simulink model "ideal_buck_boost"  (R2018a)
settings: Solver=VariableStepAuto  StartTime=0.0  StopTime=0.2  RelTol=1e-3
undefined symbols (not defined in the file): A, B, Co, current_correction_start, disturbance_Ro_enable, disturbance_Ro_time, disturbance_Vin_enable, disturbance_Vin_time, Fsw, L, opt_constant_reference, opt_equilibrium_controller, opt_pwm, opt_pwm_current_controller, opt_theorem, opt_update_equilibrium, P, pwm_limit_lower, pwm_limit_upper, pwm_period, pwm_pid_kd, pwm_pid_ki, pwm_pid_kp, pwm_pid_vc_ci, pwm_pid_vc_cp, pwm_pid_vc_vi, pwm_pid_vc_vp, pwm_sample_time, Q, R, reference_controller_initial, reference_pid_ki, reference_pid_kp, Ro, Ro_p, sys, tau, Ti, ts, Vo, Vs, Vs_p, xe
libraries: powerlib x17, simulink x12, pePwmGenerator x2
settings Model: Creator=TARCIO-FEM  LastModifiedBy=Julio-LEPO
settings OptimizationCC: EfficientMapNaN2IntZero=off
settings HardwareCC: TargetBitPerPointer=64  TargetBitPerSizeT=64  TargetBitPerPtrDiffT=64  TargetLongLongMode=on  TargetIntDivRoundTo=Zero  TargetEndianess=LittleEndian  TargetWordSize=64  TargetHWDeviceType=MATLAB Host  ProdEqTarget=off
settings CodeAppCC: MaxIdLength=128
settings GRTTargetCC: TargetLangStandard=C89/C90 (ANSI)  CombineOutputUpdateFcns=off  GRTInterface=on

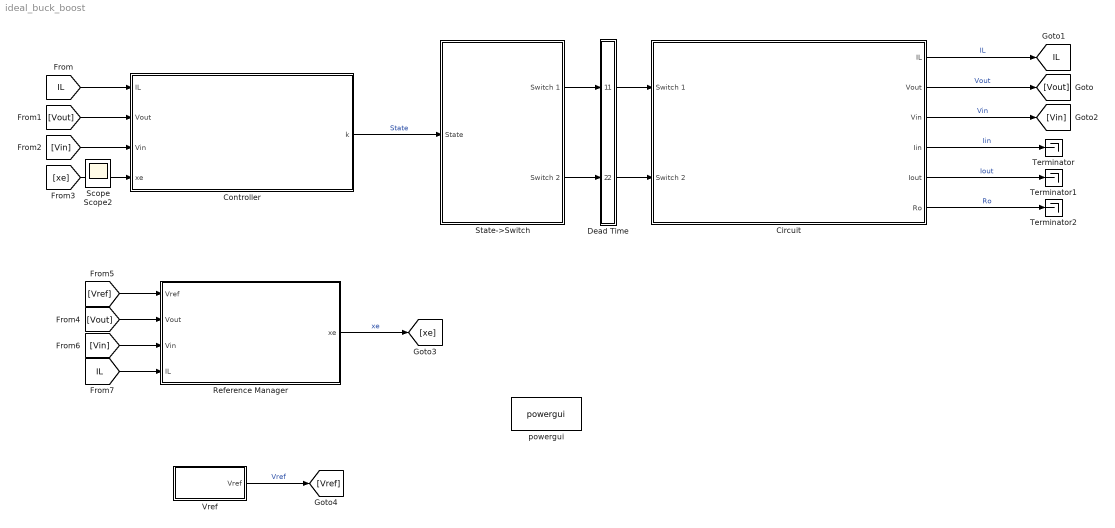
== system ideal_buck_boost ==
  Circuit : Subsystem
  Controller : Subsystem
  Dead Time : Subsystem
  Reference Manager : Subsystem
  State->Switch : Subsystem
  Terminator : Terminator
  Terminator1 : Terminator
  Terminator2 : Terminator
  Vref : Subsystem
  powergui : powerlib/powergui  Priority=1  SimulationMode=Discrete  SampleTime=Ti  frequency=60  Iterations=50  frequencyindice=0  Pbase=100e6  ErrMax=1e-4  UnitsV=kV  UnitsW=MW  buscounter=0  FunctionMessages=off  echomessages=off  EnableUseOfTLC=off  CurrentSourceSwitches=off  DisableSnubberDevices=off  DisableRonSwitches=off  DisableVfSwitches=off  DisplayEquations=off  SolverType=Tustin/Backward Euler (TBE)  Interpol=off  ExternalGateDelay=off  methode=off  Ts=100  x0status=blocks  SPID=on  SwTol=0  HookPort=off  RestoreLinks=warning  ResistiveCurrentMeasurement=off  Frange=[0:2:500]  Ylog=off  Xlog=on  ShowGrid=off  save=off  variable=ZData  structure=0  ZoomFFT=off  StartTime=0.0  cycles=1  DisplayStyle=1  fundamental=60  FreqAxis=off  MaxFrequency=1000  frequencyindicesteady=1  RmsSteady=1  display=off
  Scope : Scope
  Scope2 : Scope
  tag scope: IL=global
  wires:
  Controller/1(k) -> State->Switch/1(State)  "State"
  Circuit/3(Vin) -> [Vin]  "Vin"
  Circuit/5(Iout) -> Terminator1/1  "Iout"
  Circuit/4(Iin) -> Terminator/1  "Iin"
  Circuit/2(Vout) -> [Vout]  "Vout"
  Circuit/1(IL) -> [IL]  "IL"
  [Vout] -> Reference Manager/2(Vout)
  [Vref] -> Reference Manager/1(Vref)
  [Vin] -> Reference Manager/3(Vin)
  [IL] -> Reference Manager/4(IL)
  Reference Manager/1(xe) -> [xe]  "xe"
  Vref/1(Vref) -> [Vref]  "Vref"
  Circuit/6(Ro) -> Terminator2/1  "Ro"
  [Vout] -> Controller/2(Vout)
  [xe] -> Controller/4(xe)
  [Vin] -> Controller/3(Vin)
  [IL] -> Controller/1(IL)
  State->Switch/2(Switch 2) -> Dead Time/2(In2)
  State->Switch/1(Switch 1) -> Dead Time/1(In1)
  Dead Time/1(Out1) -> Circuit/1(Switch 1)
  Dead Time/2(Out2) -> Circuit/2(Switch 2)

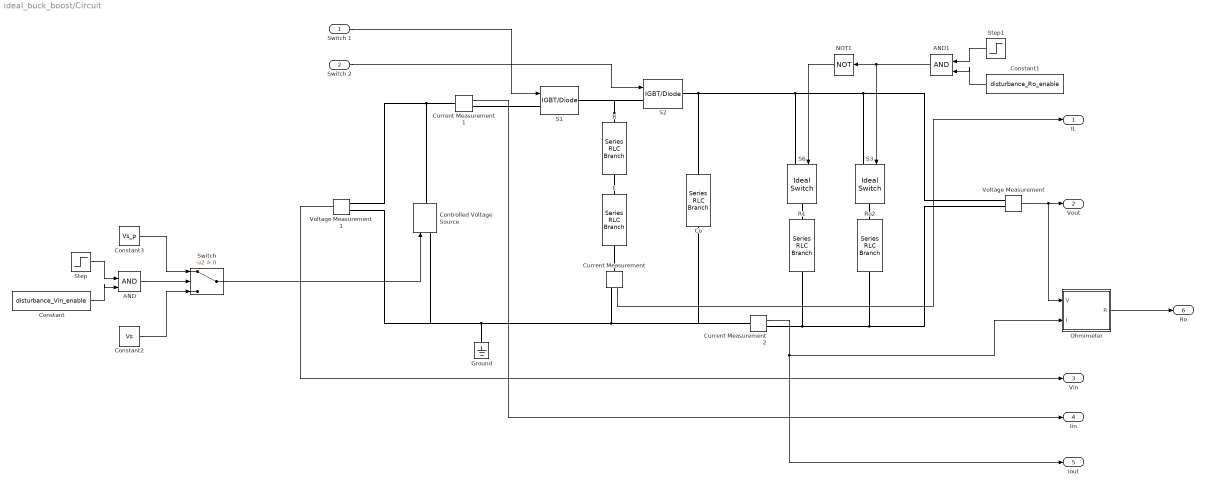
== system ideal_buck_boost/Circuit ==
  Switch 1 : Inport
  Switch 2 : Inport  Port=2
  AND : Logic  IconShape=distinctive  AllPortsSameDT=off  OutDataTypeStr=boolean
  AND1 : Logic  IconShape=distinctive  AllPortsSameDT=off  OutDataTypeStr=boolean
  Co : powerlib/Elements/Series RLC Branch  LConnTagsString=__new0  RConnTagsString=__new0  BranchType=C  Resistance=1  Inductance=L  SetiL0=off  InitialCurrent=0  Capacitance=Co  Setx0=off  InitialVoltage=0  Measurements=None
  Constant : Constant  Value=disturbance_Vin_enable
  Constant1 : Constant  Value=disturbance_Ro_enable
  Constant2 : Constant  Value=Vs
  Constant3 : Constant  Value=Vs_p
  Controlled Voltage Source : powerlib/Electrical Sources/Controlled Voltage Source  Initialize=on  Source_Type=DC  Amplitude=0  Phase=0  Frequency=0  Measurements=None
  Current Measurement : powerlib/Measurements/Current Measurement  PhasorSimulation=off  OutputType=Complex  PSBequivalent=0
  Current Measurement1 : powerlib/Measurements/Current Measurement  PhasorSimulation=off  OutputType=Complex  PSBequivalent=0
  Current Measurement2 : powerlib/Measurements/Current Measurement  PhasorSimulation=off  OutputType=Complex  PSBequivalent=0
  Ground : powerlib/Elements/Ground  LConnTagsString=a
  L : powerlib/Elements/Series RLC Branch  LConnTagsString=__new0  RConnTagsString=__new0  BranchType=L  Resistance=1  Inductance=L  SetiL0=off  InitialCurrent=0  Capacitance=1e-6  Setx0=off  InitialVoltage=0  Measurements=None
  NOT1 : Logic  Operator=NOT  IconShape=distinctive  AllPortsSameDT=off  OutDataTypeStr=boolean
  Ohmimeter : Subsystem
  R : powerlib/Elements/Series RLC Branch  LConnTagsString=__new0  RConnTagsString=__new0  BranchType=R  Resistance=R  Inductance=1e-3  SetiL0=off  InitialCurrent=0  Capacitance=1e-6  Setx0=off  InitialVoltage=0  Measurements=None
  R1 : powerlib/Elements/Series RLC Branch  LConnTagsString=__new0  RConnTagsString=__new0  BranchType=R  Resistance=Ro  Inductance=1e-3  SetiL0=off  InitialCurrent=0  Capacitance=1e-6  Setx0=off  InitialVoltage=0  Measurements=None
  Ro2 : powerlib/Elements/Series RLC Branch  LConnTagsString=__new0  RConnTagsString=__new0  BranchType=R  Resistance=Ro_p  Inductance=1e-3  SetiL0=off  InitialCurrent=0  Capacitance=1e-6  Setx0=off  InitialVoltage=0  Measurements=None
  S1 : powerlib/Power Electronics/IGBT//Diode  Ron=1e-3  Rs=1e5  Cs=inf  Measurements=off
  S2 : powerlib/Power Electronics/IGBT//Diode  Ron=1e-3  Rs=1e5  Cs=inf  Measurements=off
  S3 : powerlib/Power Electronics/Ideal Switch  Ron=0.001  Lon=0  IC=0  Rs=1e5  Cs=inf  Measurements=off
  S6 : powerlib/Power Electronics/Ideal Switch  Ron=0.001  Lon=0  IC=0  Rs=1e5  Cs=inf  Measurements=off
  Step : Step  Time=disturbance_Vin_time  SampleTime=0
  Step1 : Step  Time=disturbance_Ro_time  SampleTime=0
  Switch : Switch  Criteria=u2 > Threshold
  Voltage Measurement : powerlib/Measurements/Voltage Measurement  PhasorSimulation=off  OutputType=Complex  PSBequivalent=0
  Voltage Measurement1 : powerlib/Measurements/Voltage Measurement  PhasorSimulation=off  OutputType=Complex  PSBequivalent=0
  IL : Outport
  Vout : Outport  Port=2
  Vin : Outport  Port=3
  Iin : Outport  Port=4
  Iout : Outport  Port=5
  Ro : Outport  Port=6
  wires:
  Switch 1/1 -> S1/1
  Voltage Measurement1/1 -> Vin/1
  Current Measurement/1 -> IL/1
  Voltage Measurement/1 -> Ohmimeter/1(V), Vout/1
  Switch 2/1 -> S2/1
  AND/1 -> Switch/2
  Constant/1 -> AND/2
  Switch/1 -> Controlled Voltage Source/1
  Step/1 -> AND/1
  Constant2/1 -> Switch/3
  Constant3/1 -> Switch/1
  NOT1/1 -> S6/1
  Constant1/1 -> AND1/2
  AND1/1 -> S3/1, NOT1/1
  Step1/1 -> AND1/1
  Current Measurement1/1 -> Iin/1
  Current Measurement2/1 -> Ohmimeter/2(I), Iout/1
  Ohmimeter/1(R) -> Ro/1
  connections:
  L/LConn1 -- R/RConn1
  R/LConn1 -- S2/LConn1 -- S1/RConn1
  Current Measurement/LConn1 -- L/RConn1
  Controlled Voltage Source/RConn1 -- Current Measurement1/LConn1 -- Voltage Measurement1/LConn1
  S6/LConn1 -- S2/RConn1 -- Co/RConn1 -- S3/LConn1 -- Voltage Measurement/LConn2
  Ground/LConn1 -- Current Measurement/RConn1 -- Co/LConn1 -- Current Measurement2/LConn1 -- Voltage Measurement1/LConn2 -- Controlled Voltage Source/LConn1
  S3/RConn1 -- Ro2/LConn1
  S6/RConn1 -- R1/LConn1
  S1/LConn1 -- Current Measurement1/RConn1
  R1/RConn1 -- Current Measurement2/RConn1 -- Voltage Measurement/LConn1 -- Ro2/RConn1

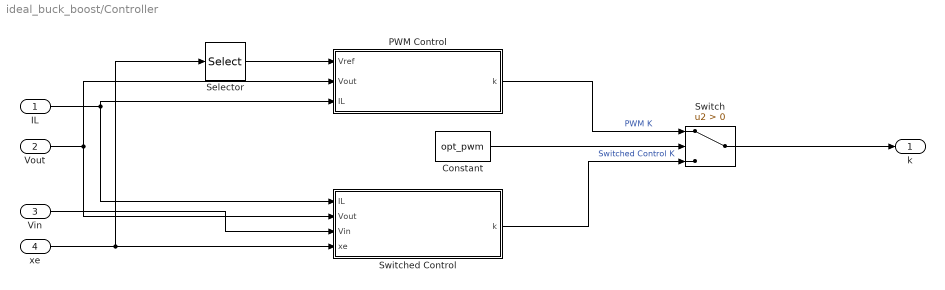
== system ideal_buck_boost/Controller ==
  IL : Inport
  Vout : Inport  Port=2
  Vin : Inport  Port=3
  xe : Inport  Port=4
  Constant : Constant  Value=opt_pwm
  PWM Control : Subsystem
  Selector : Selector  InputPortWidth=2  IndexOptions=Index vector (dialog)  Indices=[2]  OutputSizes=1
  Switch : Switch  Criteria=u2 > Threshold
  Switched Control : Subsystem
  k : Outport
  wires:
  IL/1 -> PWM Control/3(IL), Switched Control/1(IL)
  Vout/1 -> PWM Control/2(Vout), Switched Control/2(Vout)
  Vin/1 -> Switched Control/3(Vin)
  PWM Control/1(k) -> Switch/1  "PWM K"
  Switched Control/1(k) -> Switch/3  "Switched Control K"
  Constant/1 -> Switch/2
  xe/1 -> Selector/1, Switched Control/4(xe)
  Selector/1 -> PWM Control/1(Vref)
  Switch/1 -> k/1

== system ideal_buck_boost/Dead Time ==
  In1 : Inport
  In2 : Inport  Port=2
  Dead Time : Subsystem
  Dead Time1 : Subsystem
  Out1 : Outport
  Out2 : Outport  Port=2
  wires:
  Dead Time1/1(Signal Delayed) -> Out2/1
  In1/1 -> Dead Time/1(Signal)
  Dead Time/1(Signal Delayed) -> Out1/1
  In2/1 -> Dead Time1/1(Signal)

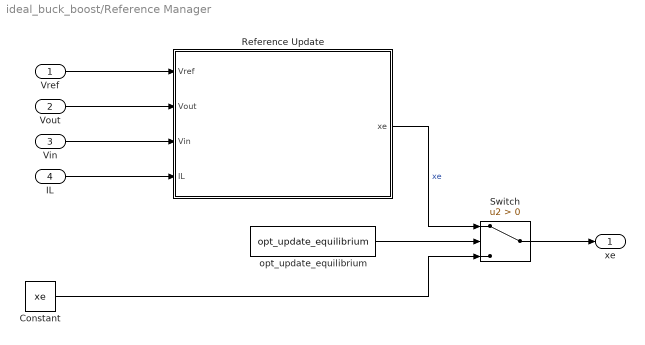
== system ideal_buck_boost/Reference Manager ==
  Vref : Inport
  Vout : Inport  Port=2
  Vin : Inport  Port=3
  IL : Inport  Port=4
  Constant : Constant  Value=xe
  Reference Update : Subsystem
  Switch : Switch  Criteria=u2 > Threshold
  opt_update_equilibrium : Constant  Value=opt_update_equilibrium
  xe : Outport
  wires:
  Vout/1 -> Reference Update/2(Vout)
  Vin/1 -> Reference Update/3(Vin)
  Vref/1 -> Reference Update/1(Vref)
  opt_update_equilibrium/1 -> Switch/2
  Switch/1 -> xe/1
  Reference Update/1(xe) -> Switch/1  "xe"
  Constant/1 -> Switch/3
  IL/1 -> Reference Update/4(IL)

== system ideal_buck_boost/State->Switch ==
  State : Inport
  Compare To Constant : simulink/Logic and Bit Operations/Compare To Constant  relop=<=  const=1.5  OutDataTypeStr=boolean
  NOT : Logic  Operator=NOT  IconShape=distinctive  AllPortsSameDT=off  OutDataTypeStr=boolean
  Switch 1 : Outport
  Switch 2 : Outport  Port=2
  wires:
  Compare To Constant/1 -> Switch 1/1, NOT/1  "Switch Signal"
  State/1 -> Compare To Constant/1
  NOT/1 -> Switch 2/1

== system ideal_buck_boost/Vref ==
  Constant Reference : Subsystem
  Switch1 : Switch  Criteria=u2 > Threshold
  Variable Reference : Subsystem
  opt_constant_reference : Constant  Value=opt_constant_reference
  Vref : Outport
  wires:
  opt_constant_reference/1 -> Switch1/2
  Switch1/1 -> Vref/1
  Variable Reference/1(Vref) -> Switch1/3
  Constant Reference/1(Vref) -> Switch1/1

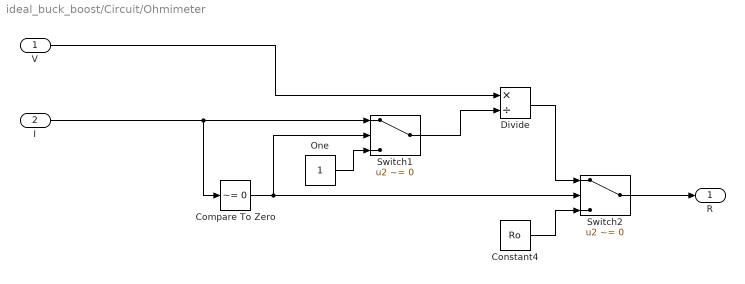
== system ideal_buck_boost/Circuit/Ohmimeter ==
  V : Inport
  I : Inport  Port=2
  Compare To Zero : simulink/Logic and Bit Operations/Compare To Zero  relop=~=  OutDataTypeStr=boolean
  Constant4 : Constant  Value=Ro
  Divide : Product  Inputs=*/
  One : Constant
  Switch1 : Switch  Criteria=u2 ~= 0
  Switch2 : Switch  Criteria=u2 ~= 0
  R : Outport
  wires:
  Compare To Zero/1 -> Switch1/2, Switch2/2
  I/1 -> Switch1/1, Compare To Zero/1
  Divide/1 -> Switch2/1
  Constant4/1 -> Switch2/3
  Switch1/1 -> Divide/2
  One/1 -> Switch1/3
  V/1 -> Divide/1
  Switch2/1 -> R/1

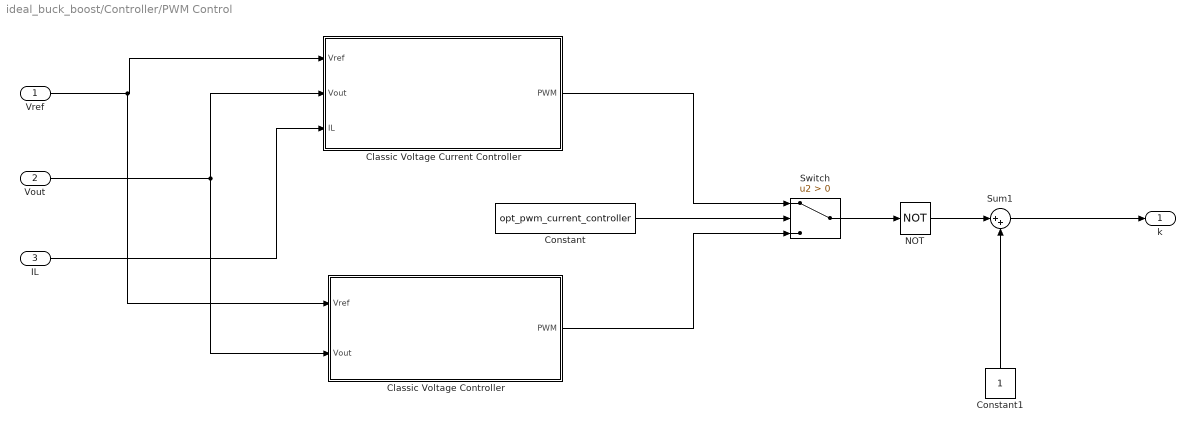
== system ideal_buck_boost/Controller/PWM Control ==
  Vref : Inport
  Vout : Inport  Port=2
  IL : Inport  Port=3
  Classic Voltage Controller : Subsystem
  Classic Voltage Current Controller : Subsystem
  Constant : Constant  Value=opt_pwm_current_controller
  Constant1 : Constant
  NOT : Logic  Operator=NOT  IconShape=distinctive  AllPortsSameDT=off  OutDataTypeStr=boolean
  Sum1 : Sum  Inputs=|++
  Switch : Switch  Criteria=u2 > Threshold
  k : Outport
  wires:
  Sum1/1 -> k/1
  NOT/1 -> Sum1/1
  Constant1/1 -> Sum1/2
  Vref/1 -> Classic Voltage Controller/1(Vref), Classic Voltage Current Controller/1(Vref)
  Vout/1 -> Classic Voltage Controller/2(Vout), Classic Voltage Current Controller/2(Vout)
  IL/1 -> Classic Voltage Current Controller/3(IL)
  Constant/1 -> Switch/2
  Switch/1 -> NOT/1
  Classic Voltage Controller/1(PWM) -> Switch/3
  Classic Voltage Current Controller/1(PWM) -> Switch/1

== system ideal_buck_boost/Controller/Switched Control ==
  IL : Inport
  Vout : Inport  Port=2
  Vin : Inport  Port=3
  xe : Inport  Port=4
  Mux : Mux  Inputs=2
  Switching Strategy : MATLAB Function  TreatAsAtomicUnit=on
  System Properties : Subsystem
  Zero-Order Hold : ZeroOrderHold  SampleTime=1/Fsw
  k : Outport
  wires:
  Vin/1 -> Switching Strategy/4(u)
  Switching Strategy/1(k) -> Zero-Order Hold/1
  System Properties/2(sys) -> Switching Strategy/2(sys)
  Mux/1 -> Switching Strategy/3(x)
  IL/1 -> Mux/1
  Vout/1 -> Mux/2
  xe/1 -> Switching Strategy/5(xe)
  Zero-Order Hold/1 -> k/1
  System Properties/1(theorem) -> Switching Strategy/1(theorem)

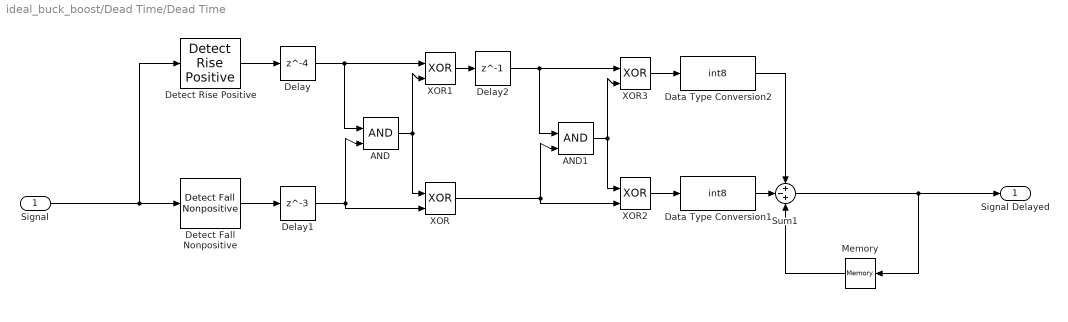
== system ideal_buck_boost/Dead Time/Dead Time ==
  Signal : Inport
  AND : Logic  IconShape=distinctive  AllPortsSameDT=off  OutDataTypeStr=boolean
  AND1 : Logic  IconShape=distinctive  AllPortsSameDT=off  OutDataTypeStr=boolean
  Data Type Conversion1 : DataTypeConversion  OutDataTypeStr=int8
  Data Type Conversion2 : DataTypeConversion  OutDataTypeStr=int8
  Delay : Delay  DelayLength=4
  Delay1 : Delay  DelayLength=3
  Delay2 : Delay  DelayLength=1
  Detect Fall Nonpositive : simulink/Logic and Bit Operations/Detect Fall Nonpositive  vinit=0  OutDataTypeStr=boolean
      settings: SourceProductName=Simulink  SourceProductBaseCode=SL
  Detect Rise Positive : simulink/Logic and Bit Operations/Detect Rise Positive  vinit=0  OutDataTypeStr=boolean
  Memory : Memory  InheritSampleTime=on  LinearizeAsDelay=on
  Sum1 : Sum  Inputs=+-+
  XOR{,1..3} (4 alike) : Logic  Operator=XOR  IconShape=distinctive  AllPortsSameDT=off  OutDataTypeStr=boolean
  Signal Delayed : Outport
  wires:
  Sum1/1 -> Memory/1, Signal Delayed/1
  Data Type Conversion1/1 -> Sum1/2
  Memory/1 -> Sum1/3
  Signal/1 -> Detect Rise Positive/1, Detect Fall Nonpositive/1
  Data Type Conversion2/1 -> Sum1/1
  Detect Fall Nonpositive/1 -> Delay1/1
  Detect Rise Positive/1 -> Delay/1
  Delay1/1 -> XOR/2, AND/2
  Delay/1 -> XOR1/1, AND/1
  XOR1/1 -> Delay2/1
  AND/1 -> XOR1/2, XOR/1
  Delay2/1 -> XOR3/1, AND1/1
  AND1/1 -> XOR3/2, XOR2/1
  XOR/1 -> XOR2/2, AND1/2
  XOR3/1 -> Data Type Conversion2/1
  XOR2/1 -> Data Type Conversion1/1

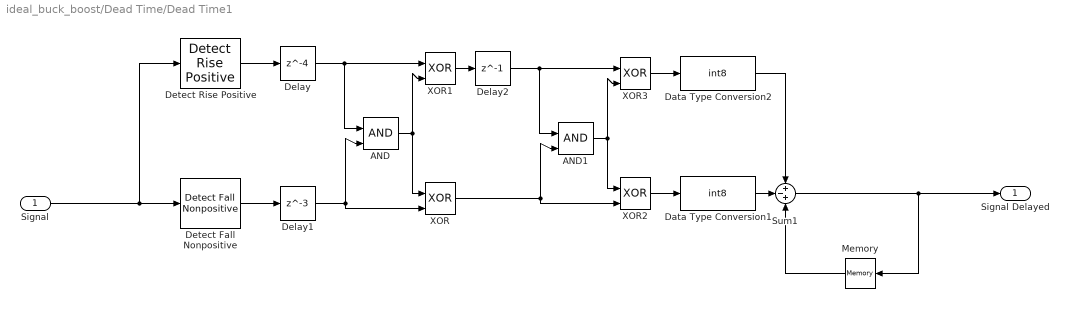
== system ideal_buck_boost/Dead Time/Dead Time1 ==
  Signal : Inport
  AND : Logic  IconShape=distinctive  AllPortsSameDT=off  OutDataTypeStr=boolean
  AND1 : Logic  IconShape=distinctive  AllPortsSameDT=off  OutDataTypeStr=boolean
  Data Type Conversion1 : DataTypeConversion  OutDataTypeStr=int8
  Data Type Conversion2 : DataTypeConversion  OutDataTypeStr=int8
  Delay : Delay  DelayLength=4
  Delay1 : Delay  DelayLength=3
  Delay2 : Delay  DelayLength=1
  Detect Fall Nonpositive : simulink/Logic and Bit Operations/Detect Fall Nonpositive  vinit=0  OutDataTypeStr=boolean
      settings: SourceProductName=Simulink  SourceProductBaseCode=SL
  Detect Rise Positive : simulink/Logic and Bit Operations/Detect Rise Positive  vinit=0  OutDataTypeStr=boolean
  Memory : Memory  InheritSampleTime=on  LinearizeAsDelay=on
  Sum1 : Sum  Inputs=+-+
  XOR{,1..3} (4 alike) : Logic  Operator=XOR  IconShape=distinctive  AllPortsSameDT=off  OutDataTypeStr=boolean
  Signal Delayed : Outport
  wires:
  Sum1/1 -> Memory/1, Signal Delayed/1
  Data Type Conversion1/1 -> Sum1/2
  Memory/1 -> Sum1/3
  Signal/1 -> Detect Rise Positive/1, Detect Fall Nonpositive/1
  Data Type Conversion2/1 -> Sum1/1
  Detect Fall Nonpositive/1 -> Delay1/1
  Detect Rise Positive/1 -> Delay/1
  Delay1/1 -> XOR/2, AND/2
  Delay/1 -> XOR1/1, AND/1
  XOR1/1 -> Delay2/1
  AND/1 -> XOR1/2, XOR/1
  Delay2/1 -> XOR3/1, AND1/1
  AND1/1 -> XOR3/2, XOR2/1
  XOR/1 -> XOR2/2, AND1/2
  XOR3/1 -> Data Type Conversion2/1
  XOR2/1 -> Data Type Conversion1/1

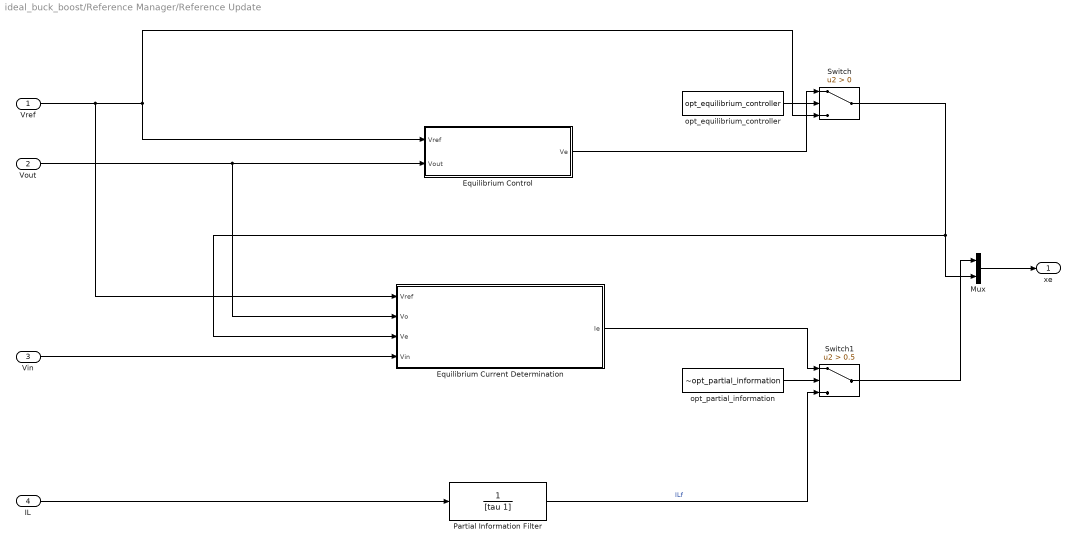
== system ideal_buck_boost/Reference Manager/Reference Update ==
  Vref : Inport
  Vout : Inport  Port=2
  Vin : Inport  Port=3
  IL : Inport  Port=4
  Equilibrium Control : Subsystem
  Equilibrium Current Determination : Subsystem
  Mux : Mux  Inputs=2
  Partial Information Filter : TransferFcn  Denominator=[tau 1]
  Switch : Switch  Criteria=u2 > Threshold
  Switch1 : Switch  Criteria=u2 > Threshold  Threshold=0.5
  opt_equilibrium_controller : Constant  Value=opt_equilibrium_controller
  opt_partial_information : Constant  Value=~opt_partial_information
  xe : Outport
  wires:
  Vref/1 -> Equilibrium Current Determination/1(Vref), Equilibrium Control/1(Vref), Switch/3
  Mux/1 -> xe/1
  opt_equilibrium_controller/1 -> Switch/2
  Switch/1 -> Equilibrium Current Determination/3(Ve), Mux/2
  Switch1/1 -> Mux/1
  opt_partial_information/1 -> Switch1/2
  Partial Information Filter/1 -> Switch1/3  "ILf"
  IL/1 -> Partial Information Filter/1
  Vout/1 -> Equilibrium Current Determination/2(Vo), Equilibrium Control/2(Vout)
  Equilibrium Control/1(Ve) -> Switch/1
  Vin/1 -> Equilibrium Current Determination/4(Vin)
  Equilibrium Current Determination/1(Ie) -> Switch1/1

== system ideal_buck_boost/Vref/Constant Reference ==
  Constant : Constant  Value=xe
  Selector : Selector  InputPortWidth=2  IndexOptions=Index vector (dialog)  Indices=[2]  OutputSizes=1
  Vref : Outport
  wires:
  Constant/1 -> Selector/1
  Selector/1 -> Vref/1

== system ideal_buck_boost/Vref/Variable Reference ==
  0 : Gain
  Ramp2 : simulink/Sources/Ramp  slope=Vo/ts  start=0  InitialOutput=0
  Ramp3 : simulink/Sources/Ramp  slope=Vo/ts  start=ts  InitialOutput=0
  Rate Transition10 : RateTransition  OutPortSampleTimeOpt=Inherit  OutPortSampleTime=Ts
  Sum1 : Sum  Inputs=++-
  Vdc_Ref : Step  Time=0.3  After=10  SampleTime=0
  Vref : Outport
  wires:
  Ramp2/1 -> Sum1/2
  Sum1/1 -> 0/1
  Vdc_Ref/1 -> Sum1/1
  Ramp3/1 -> Sum1/3
  0/1 -> Rate Transition10/1
  Rate Transition10/1 -> Vref/1

== system ideal_buck_boost/Controller/PWM Control/Classic Voltage Controller ==
  Vref : Inport
  Vout : Inport  Port=2
  PID Controller : simulink/Continuous/PID Controller  Controller=PI  TimeDomain=Discrete-time  SampleTime=pwm_period  IntegratorMethod=Forward Euler  FilterMethod=Forward Euler  Form=Parallel  UseFilter=on  ControllerParametersSource=internal  P=pwm_pid_kp  I=pwm_pid_ki  D=pwm_pid_kd  N=100  InitialConditionSource=internal  InitialConditionForIntegrator=0  InitialConditionForFilter=0  ExternalReset=none  LimitOutput=off  UpperSaturationLimit=inf  LowerSaturationLimit=-inf  LinearizeAsGain=on  AntiWindupMode=none  Kb=1  TrackingMode=off  Kt=1  PParamMin=[]  PParamMax=[]  IParamMin=[]  IParamMax=[]  DParamMin=[]  DParamMax=[]  NParamMin=[]  NParamMax=[]  KbParamMin=[]  KbParamMax=[]  KtParamMin=[]  KtParamMax=[]  POutMin=[]  POutMax=[]  IOutMin=[]  IOutMax=[]  DOutMin=[]  DOutMax=[]  NOutMin=[]  NOutMax=[]  KbOutMin=[]  KbOutMax=[]  KtOutMin=[]  KtOutMax=[]  IntegratorOutMin=[]  IntegratorOutMax=[]  FilterOutMin=[]  FilterOutMax=[]  SumOutMin=[]  SumOutMax=[]  SumI1OutMin=[]  SumI1OutMax=[]  SumI2OutMin=[]  SumI2OutMax=[]  SumI3OutMin=[]  SumI3OutMax=[]  SumDOutMin=[]  SumDOutMax=[]  SaturationOutMin=[]  SaturationOutMax=[]  IntegratorContinuousStateAttributes=''  IntegratorStateMustResolveToSignalObject=off  IntegratorRTWStateStorageClass=Auto  FilterContinuousStateAttributes=''  FilterStateMustResolveToSignalObject=off  FilterRTWStateStorageClass=Auto  DifferentiatorICPrevScaledInput=0  DifferentiatorOutMin=[]  DifferentiatorOutMax=[]  FilterDiffOutCoefMin=[]  FilterDiffOutCoefMax=[]  SumDenOutMin=[]  SumDenOutMax=[]  SumNumOutMin=[]  SumNumOutMax=[]  ReciprocalOutMin=[]  ReciprocalOutMax=[]  DivideOutMin=[]  DivideOutMax=[]  TunerSelectOption=Transfer Function Based (PID Tuner App)
  PWM Generator : pePwmGenerator/PWM Generator  CarrCount=Up  Tper=pwm_period  Ts=pwm_sample_time
  Saturation : Saturate  UpperLimit=pwm_limit_upper  LowerLimit=pwm_limit_lower
  Sum : Sum  Inputs=|+-
  PWM : Outport
  wires:
  Saturation/1 -> PWM Generator/1  "PWM Duty Cycle"
  PWM Generator/1 -> PWM/1
  PID Controller/1 -> Saturation/1
  Sum/1 -> PID Controller/1
  Vref/1 -> Sum/1
  Vout/1 -> Sum/2

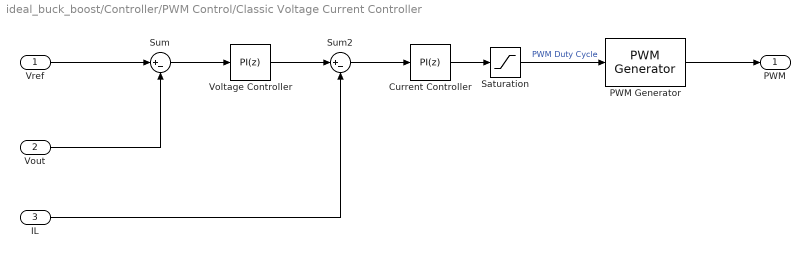
== system ideal_buck_boost/Controller/PWM Control/Classic Voltage Current Controller ==
  Vref : Inport
  Vout : Inport  Port=2
  IL : Inport  Port=3
  Current Controller : simulink/Continuous/PID Controller  Controller=PI  TimeDomain=Discrete-time  SampleTime=pwm_period  IntegratorMethod=Forward Euler  FilterMethod=Forward Euler  Form=Parallel  UseFilter=on  ControllerParametersSource=internal  P=pwm_pid_vc_cp  I=pwm_pid_vc_ci  D=pwm_pid_kd  N=100  InitialConditionSource=internal  InitialConditionForIntegrator=0  InitialConditionForFilter=0  ExternalReset=none  LimitOutput=off  UpperSaturationLimit=inf  LowerSaturationLimit=-inf  LinearizeAsGain=on  AntiWindupMode=none  Kb=1  TrackingMode=off  Kt=1  PParamMin=[]  PParamMax=[]  IParamMin=[]  IParamMax=[]  DParamMin=[]  DParamMax=[]  NParamMin=[]  NParamMax=[]  KbParamMin=[]  KbParamMax=[]  KtParamMin=[]  KtParamMax=[]  POutMin=[]  POutMax=[]  IOutMin=[]  IOutMax=[]  DOutMin=[]  DOutMax=[]  NOutMin=[]  NOutMax=[]  KbOutMin=[]  KbOutMax=[]  KtOutMin=[]  KtOutMax=[]  IntegratorOutMin=[]  IntegratorOutMax=[]  FilterOutMin=[]  FilterOutMax=[]  SumOutMin=[]  SumOutMax=[]  SumI1OutMin=[]  SumI1OutMax=[]  SumI2OutMin=[]  SumI2OutMax=[]  SumI3OutMin=[]  SumI3OutMax=[]  SumDOutMin=[]  SumDOutMax=[]  SaturationOutMin=[]  SaturationOutMax=[]  IntegratorContinuousStateAttributes=''  IntegratorStateMustResolveToSignalObject=off  IntegratorRTWStateStorageClass=Auto  FilterContinuousStateAttributes=''  FilterStateMustResolveToSignalObject=off  FilterRTWStateStorageClass=Auto  DifferentiatorICPrevScaledInput=0  DifferentiatorOutMin=[]  DifferentiatorOutMax=[]  FilterDiffOutCoefMin=[]  FilterDiffOutCoefMax=[]  SumDenOutMin=[]  SumDenOutMax=[]  SumNumOutMin=[]  SumNumOutMax=[]  ReciprocalOutMin=[]  ReciprocalOutMax=[]  DivideOutMin=[]  DivideOutMax=[]  TunerSelectOption=Transfer Function Based (PID Tuner App)
  PWM Generator : pePwmGenerator/PWM Generator  CarrCount=Up  Tper=pwm_period  Ts=pwm_sample_time
  Saturation : Saturate  UpperLimit=pwm_limit_upper  LowerLimit=pwm_limit_lower
  Sum : Sum  Inputs=|+-
  Sum2 : Sum  Inputs=|+-
  Voltage Controller : simulink/Continuous/PID Controller  Controller=PI  TimeDomain=Discrete-time  SampleTime=pwm_period  IntegratorMethod=Forward Euler  FilterMethod=Forward Euler  Form=Parallel  UseFilter=on  ControllerParametersSource=internal  P=pwm_pid_vc_vp  I=pwm_pid_vc_vi  D=0  N=100  InitialConditionSource=internal  InitialConditionForIntegrator=0  InitialConditionForFilter=0  ExternalReset=none  LimitOutput=off  UpperSaturationLimit=inf  LowerSaturationLimit=-inf  LinearizeAsGain=on  AntiWindupMode=none  Kb=1  TrackingMode=off  Kt=1  PParamMin=[]  PParamMax=[]  IParamMin=[]  IParamMax=[]  DParamMin=[]  DParamMax=[]  NParamMin=[]  NParamMax=[]  KbParamMin=[]  KbParamMax=[]  KtParamMin=[]  KtParamMax=[]  POutMin=[]  POutMax=[]  IOutMin=[]  IOutMax=[]  DOutMin=[]  DOutMax=[]  NOutMin=[]  NOutMax=[]  KbOutMin=[]  KbOutMax=[]  KtOutMin=[]  KtOutMax=[]  IntegratorOutMin=[]  IntegratorOutMax=[]  FilterOutMin=[]  FilterOutMax=[]  SumOutMin=[]  SumOutMax=[]  SumI1OutMin=[]  SumI1OutMax=[]  SumI2OutMin=[]  SumI2OutMax=[]  SumI3OutMin=[]  SumI3OutMax=[]  SumDOutMin=[]  SumDOutMax=[]  SaturationOutMin=[]  SaturationOutMax=[]  IntegratorContinuousStateAttributes=''  IntegratorStateMustResolveToSignalObject=off  IntegratorRTWStateStorageClass=Auto  FilterContinuousStateAttributes=''  FilterStateMustResolveToSignalObject=off  FilterRTWStateStorageClass=Auto  DifferentiatorICPrevScaledInput=0  DifferentiatorOutMin=[]  DifferentiatorOutMax=[]  FilterDiffOutCoefMin=[]  FilterDiffOutCoefMax=[]  SumDenOutMin=[]  SumDenOutMax=[]  SumNumOutMin=[]  SumNumOutMax=[]  ReciprocalOutMin=[]  ReciprocalOutMax=[]  DivideOutMin=[]  DivideOutMax=[]  TunerSelectOption=Transfer Function Based (PID Tuner App)
  PWM : Outport
  wires:
  Sum2/1 -> Current Controller/1
  Sum/1 -> Voltage Controller/1
  Vout/1 -> Sum/2
  Voltage Controller/1 -> Sum2/1
  IL/1 -> Sum2/2
  Current Controller/1 -> Saturation/1
  Vref/1 -> Sum/1
  Saturation/1 -> PWM Generator/1  "PWM Duty Cycle"
  PWM Generator/1 -> PWM/1

== system ideal_buck_boost/Controller/Switched Control/System Properties ==
  Bus Creator : BusCreator  Inputs=5  OutDataTypeStr=Bus: SystemDataBus
  Constant : Constant  Value=A  VectorParams1D=off
  Constant1 : Constant  Value=B  VectorParams1D=off
  Constant2 : Constant  Value=P  VectorParams1D=off
  Constant3 : Constant  Value=Q  VectorParams1D=off
  Constant5 : Constant  Value=sys.N
  Constant6 : Constant  Value=opt_theorem
  theorem : Outport
  sys : Outport  Port=2
  wires:
  Bus Creator/1 -> sys/1
  Constant2/1 -> Bus Creator/3  "P"
  Constant1/1 -> Bus Creator/2  "B"
  Constant/1 -> Bus Creator/1  "A"
  Constant3/1 -> Bus Creator/4  "Q"
  Constant5/1 -> Bus Creator/5  "N"
  Constant6/1 -> theorem/1

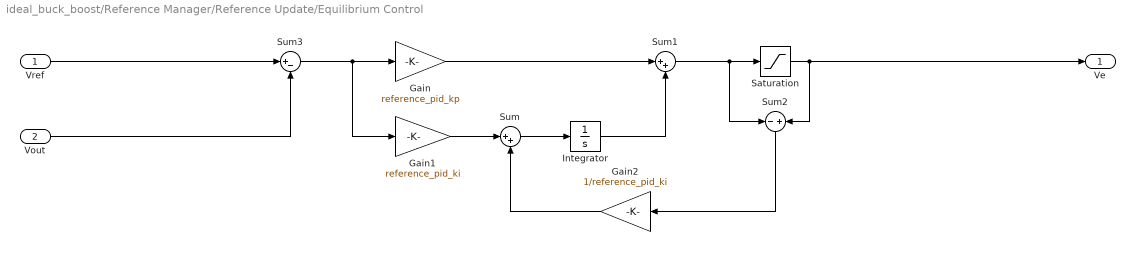
== system ideal_buck_boost/Reference Manager/Reference Update/Equilibrium Control ==
  Vref : Inport
  Vout : Inport  Port=2
  Gain : Gain  Gain=reference_pid_kp
  Gain1 : Gain  Gain=reference_pid_ki
  Gain2 : Gain  Gain=1/reference_pid_ki
  Integrator : Integrator  InitialCondition=reference_controller_initial
  Saturation : Saturate  UpperLimit=400  LowerLimit=0
  Sum : Sum  Inputs=|++
  Sum1 : Sum  Inputs=|++
  Sum2 : Sum  Inputs=-|+
  Sum3 : Sum  Inputs=|+-
  Ve : Outport
  wires:
  Sum1/1 -> Sum2/1, Saturation/1
  Sum/1 -> Integrator/1
  Gain1/1 -> Sum/1
  Integrator/1 -> Sum1/2
  Vout/1 -> Sum3/2
  Sum3/1 -> Gain1/1, Gain/1
  Gain/1 -> Sum1/1
  Gain2/1 -> Sum/2
  Saturation/1 -> Ve/1, Sum2/2
  Sum2/1 -> Gain2/1
  Vref/1 -> Sum3/1

== system ideal_buck_boost/Reference Manager/Reference Update/Equilibrium Current Determination ==
  Vref : Inport
  Vo : Inport  Port=2
  Ve : Inport  Port=3
  Vin : Inport  Port=4
  Current Correction : Subsystem
  Current Estimation : Subsystem
  Switch2 : Switch  Criteria=u2 > Threshold  Threshold=0.5
  opt_current_correction : Constant  Value=~opt_current_correction
  Ie : Outport
  wires:
  Ve/1 -> Current Estimation/1(Ve)
  Current Correction/1(Ie) -> Switch2/3
  Switch2/1 -> Ie/1
  opt_current_correction/1 -> Switch2/2
  Current Estimation/1(Ie) -> Current Correction/1(IL_e), Switch2/1
  Vref/1 -> Current Correction/2(Vref)
  Vin/1 -> Current Estimation/2(Vin)
  Vo/1 -> Current Correction/3(Vo)

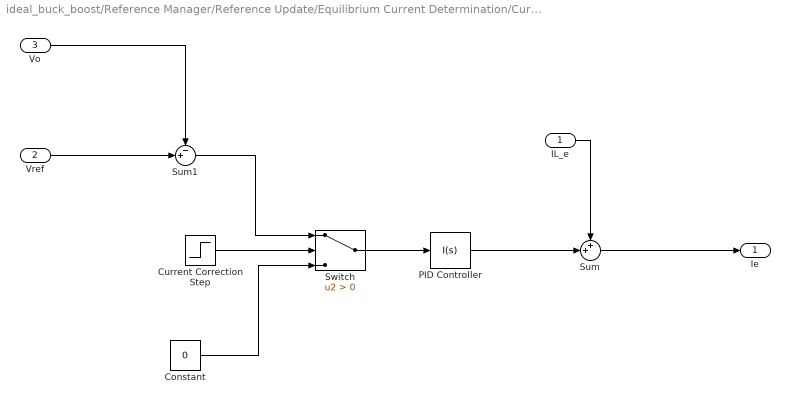
== system ideal_buck_boost/Reference Manager/Reference Update/Equilibrium Current Determination/Current Correction ==
  IL_e : Inport
  Vref : Inport  Port=2
  Vo : Inport  Port=3
  Constant : Constant  Value=0
  Current Correction Step : Step  Time=current_correction_start  SampleTime=0
  PID Controller : simulink/Continuous/PID Controller  Controller=I  TimeDomain=Continuous-time  SampleTime=-1  IntegratorMethod=Forward Euler  FilterMethod=Forward Euler  Form=Parallel  UseFilter=on  ControllerParametersSource=internal  P=0  I=5  D=0  N=100  InitialConditionSource=internal  InitialConditionForIntegrator=0  InitialConditionForFilter=0  ExternalReset=none  LimitOutput=off  UpperSaturationLimit=inf  LowerSaturationLimit=-inf  LinearizeAsGain=on  AntiWindupMode=none  Kb=1  TrackingMode=off  Kt=1  PParamMin=[]  PParamMax=[]  IParamMin=[]  IParamMax=[]  DParamMin=[]  DParamMax=[]  NParamMin=[]  NParamMax=[]  KbParamMin=[]  KbParamMax=[]  KtParamMin=[]  KtParamMax=[]  POutMin=[]  POutMax=[]  IOutMin=[]  IOutMax=[]  DOutMin=[]  DOutMax=[]  NOutMin=[]  NOutMax=[]  KbOutMin=[]  KbOutMax=[]  KtOutMin=[]  KtOutMax=[]  IntegratorOutMin=[]  IntegratorOutMax=[]  FilterOutMin=[]  FilterOutMax=[]  SumOutMin=[]  SumOutMax=[]  SumI1OutMin=[]  SumI1OutMax=[]  SumI2OutMin=[]  SumI2OutMax=[]  SumI3OutMin=[]  SumI3OutMax=[]  SumDOutMin=[]  SumDOutMax=[]  SaturationOutMin=[]  SaturationOutMax=[]  IntegratorContinuousStateAttributes=''  IntegratorStateMustResolveToSignalObject=off  IntegratorRTWStateStorageClass=Auto  FilterContinuousStateAttributes=''  FilterStateMustResolveToSignalObject=off  FilterRTWStateStorageClass=Auto  DifferentiatorICPrevScaledInput=0  DifferentiatorOutMin=[]  DifferentiatorOutMax=[]  FilterDiffOutCoefMin=[]  FilterDiffOutCoefMax=[]  SumDenOutMin=[]  SumDenOutMax=[]  SumNumOutMin=[]  SumNumOutMax=[]  ReciprocalOutMin=[]  ReciprocalOutMax=[]  DivideOutMin=[]  DivideOutMax=[]  TunerSelectOption=Transfer Function Based (PID Tuner App)
  Sum : Sum  Inputs=++|
  Sum1 : Sum  Inputs=-+|
  Switch : Switch  Criteria=u2 > Threshold
  Ie : Outport
  wires:
  Vo/1 -> Sum1/1
  PID Controller/1 -> Sum/2
  Sum/1 -> Ie/1
  Vref/1 -> Sum1/2
  IL_e/1 -> Sum/1
  Switch/1 -> PID Controller/1
  Current Correction Step/1 -> Switch/2
  Sum1/1 -> Switch/1
  Constant/1 -> Switch/3

== system ideal_buck_boost/Reference Manager/Reference Update/Equilibrium Current Determination/Current Estimation ==
  Ve : Inport
  Vin : Inport  Port=2
  Buck-Boost Equilibrium Current : MATLAB Function  TreatAsAtomicUnit=on
  Constant : Constant  Value=R
  Constant1 : Constant  Value=Ro
  Ie : Outport
  wires:
  Buck-Boost Equilibrium Current/1(I) -> Ie/1
  Constant/1 -> Buck-Boost Equilibrium Current/3(R)
  Vin/1 -> Buck-Boost Equilibrium Current/2(Vin)
  Ve/1 -> Buck-Boost Equilibrium Current/1(Ve)
  Constant1/1 -> Buck-Boost Equilibrium Current/4(Ro)

== matlab function ideal_buck_boost/Controller/Switched Control/Switching Strategy ==
  data: theorem input; sys input; x input; u input; k output; xe input
function k = switching_strategy(theorem, sys, x, u, xe)
    qsi = x - xe;
    sig = zeros(sys.N,1);
    
    for i=1:sys.N
        switch(theorem)
            case 1
                sig(i) = qsi'*(sys.Q(:,:,i)*qsi + 2*sys.P*(sys.A(:,:,i)*x + sys.B(:,:,i)*u));
            case 2
                sig(i) = qsi'*sys.P*(sys.A(:,:,i)*xe + sys.B(:,:,i)*u);
        end
    end
    [~, k] = min(sig);
end

== matlab function ideal_buck_boost/Reference Manager/Reference Update/Equilibrium Current Determination/Current Estimation/Buck-Boost Equilibrium Current ==
  data: Ve input; I output; Vin input; R input; Ro input
function I = EquilibriumCurrent(Ve, Vin, R, Ro)
    I = Vin/(2*R) - sqrt( Vin^2/(4*R^2) - Ve*(Ve+Vin)/(R*Ro) );
end
